simulink model "rotary_system"  (R2023b)
settings: Solver=ode4  StartTime=0.0  StopTime=0.3  FixedStep=1e-6  MaxStep=1e-5  RelTol=1e-6
InitFcn:
  | %% Parameters
  | 
  | param = struct();
  | 
  | % Volume of chambers
  | param.V1_0 = 2e-3;
  | param.V2_0 = 20e-6;
  | 
  | % Pressure rails
  | param.P_H = 20e6;
  | param.P_M = 10e6;
  | 
  | % Valve things
  | param.max_Avt = 0.5*0.25*pi*(20e-3)^2;
  | param.Cd = 0.6;
  | 
  | % Fluid properties
  | param.beta = 1.8e9;
  | param.rho = 870;
  | 
  | % Electric motor stuff
  | param.Kt = 70.5e-3;
  | param.Ke = 70.5e-3;
  | param.J_elec = 140e-7;
  | 
  | % Pump things
  | param.J_hyd = 53000e-7;
  | param.hyd_D = 6.29e-6;    % In cc/rev
settings Model: Creator=user  LastModifiedBy=user

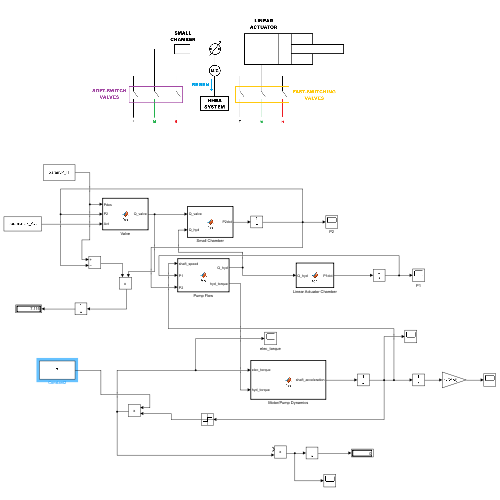
[thumbnail: Simulink's stored preview of the top-level diagram]
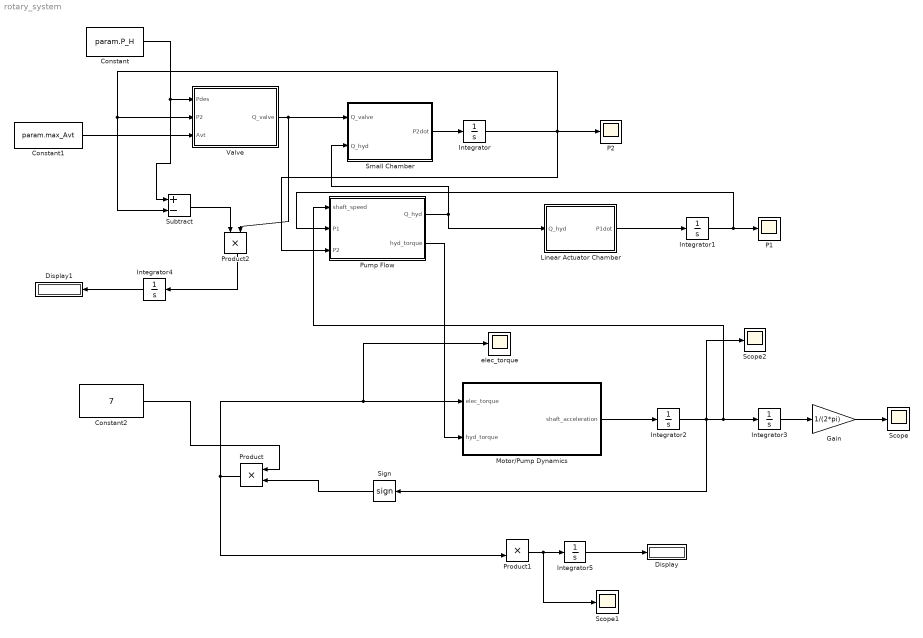
== system rotary_system ==
  Constant : Constant  Value=param.P_H
  Constant1 : Constant  Value=param.max_Avt
  Constant2 : Constant  Value=7
  Display : Display
  Display1 : Display
  Gain : Gain  Gain=1/(2*pi)
  Integrator : Integrator  InitialCondition=param.P_M
  Integrator1 : Integrator  InitialCondition=param.P_M
  Integrator{2..5} (4 alike) : Integrator
  Linear Actuator Chamber : MATLAB Function  TreatAsAtomicUnit=on
  Motor/Pump Dynamics : MATLAB Function  TreatAsAtomicUnit=on
  P1 : Scope
  P2 : Scope
  Product : Product
  Product1 : Product
  Product2 : Product
  Pump Flow : MATLAB Function  TreatAsAtomicUnit=on
  Scope : Scope
  Scope1 : Scope
  Scope2 : Scope
  Sign : Signum
  Small Chamber : MATLAB Function  TreatAsAtomicUnit=on
  Subtract : Sum  Inputs=+-
  Valve : MATLAB Function  TreatAsAtomicUnit=on
  elec_torque : Scope
  wires:
  Small Chamber/1(P2dot) -> Integrator/1
  Linear Actuator Chamber/1(P1dot) -> Integrator1/1
  Pump Flow/1(Q_hyd) -> Linear Actuator Chamber/1(Q_hyd), Small Chamber/2(Q_hyd)
  Valve/1(Q_valve) -> Product2/2, Small Chamber/1(Q_valve)
  Constant/1 -> Subtract/1, Valve/1(Pdes)
  Constant1/1 -> Valve/3(Avt)
  Integrator/1 -> Pump Flow/3(P2), P2/1, Subtract/2, Valve/2(P2)
  Integrator1/1 -> Pump Flow/2(P1), P1/1
  Motor/Pump Dynamics/1(shaft_acceleration) -> Integrator2/1
  Integrator2/1 -> Sign/1, Scope2/1, Integrator3/1, Pump Flow/1(shaft_speed)
  Pump Flow/2(hyd_torque) -> Motor/Pump Dynamics/2(hyd_torque)
  Integrator3/1 -> Gain/1
  Gain/1 -> Scope/1
  Sign/1 -> Product/2
  Constant2/1 -> Product/1
  Product/1 -> elec_torque/1, Motor/Pump Dynamics/1(elec_torque), Product1/2
  Product1/1 -> Scope1/1, Integrator5/1
  Subtract/1 -> Product2/1
  Product2/1 -> Integrator4/1
  Integrator4/1 -> Display1/1
  Integrator5/1 -> Display/1

== matlab function rotary_system/Small Chamber ==
  data: P2dot output; param parameter; Q_valve input; Q_hyd input
function P2dot = fcn(param, Q_valve, Q_hyd)

P2dot = (param.beta/param.V2_0)*(Q_valve - Q_hyd);

== matlab function rotary_system/Valve ==
  data: Q_valve output; Pdes input; P2 input; Avt input; param parameter
function Q_valve = fcn(Pdes, P2, Avt, param)

Q_valve = param.Cd*Avt*sqrt((2/param.rho)*abs(Pdes-P2))*sign(Pdes-P2);

== matlab function rotary_system/Pump Flow ==
  data: Q_hyd output; param parameter; shaft_speed input; P1 input; P2 input; hyd_torque output
function [Q_hyd, hyd_torque] = fcn(param, shaft_speed, P1, P2)

Q_hyd = (param.hyd_D/(2*pi))*shaft_speed;

hyd_torque = (param.hyd_D/(2*pi))*(P2 - P1);

% Q_pump = (param.hyd_D/(2*pi))*shaft_speed;

== matlab function rotary_system/Linear Actuator Chamber ==
  data: P1dot output; param parameter; Q_hyd input
function P1dot = fcn(param, Q_hyd)

P1dot = (param.beta/param.V1_0)*Q_hyd;

== matlab function rotary_system/Motor//Pump Dynamics ==
  data: shaft_acceleration output; param parameter; elec_torque input; hyd_torque input
function shaft_acceleration = fcn(param, elec_torque, hyd_torque)

shaft_acceleration = (1/(param.J_hyd+param.J_elec))*(hyd_torque - elec_torque);
